simulink model "mrefrobotarm_modified_previous_y_previous_u_previous_ref_pert_2"  (R2018b)
settings: Solver=FixedStepAuto  StartTime=0.0  StopTime=60  RelTol=1e-3  AbsTol=1e-6
undefined symbols (not defined in the file or in its folder): cc, options
libraries: neural x858, simulink x1
(part 18 of 32)

== system mrefrobotarm_modified_previous_y_previous_u_previous_ref_pert_2/m=0 sd=0.2/Layer 3/Delays 1 ==
  "p{3}" : Inport  PortDimensions=30
      mask Display: e = 0.06;c1 = [120 230 180]/255;c2 = ([120 230 180]+0)/(256+128);c3 = ([120 230 180]+128)/(256+128);patch([0 1 1 0],[0 0 1 1],c1);patch([0 1 1 1-e 1-e 0+e],[0 0 1 1-e 0+e 0+e],c2);patch([0 0 1 1-e 0+e 0+e],[0 1 1 1-e 1-e 0+e],c3);plot([0 1 1 0 0],[0 0 1 1 0]);
  mux : Mux  Inputs=1
      mask Display: e = 0.06;c1 = [120 150 230]/255;c2 = ([120 150 230]+0)/383;c3 = ([120 150 230]+128)/383;patch([0 1 1 0],[0 0 1 1],c1);patch([0 1 1 1-e 1-e 0+e],[0 0 1 1-e 0+e 0+e],c2);patch([0 0 1 1-e 0+e 0+e],[0 1 1 1-e 1-e 0+e],c3);plot([0 1 1 0 0],[0 0 1 1 0]);disp('Mux')
  "pd{3,2}" : Outport
      mask Display: e = 0.06;c1 = [120 230 180]/255;c2 = ([120 230 180]+0)/(256+128);c3 = ([120 230 180]+128)/(256+128);patch([0 1 1 0],[0 0 1 1],c1);patch([0 1 1 1-e 1-e 0+e],[0 0 1 1-e 0+e 0+e],c2);patch([0 0 1 1-e 0+e 0+e],[0 1 1 1-e 1-e 0+e],c3);plot([0 1 1 0 0],[0 0 1 1 0]);
  wires:
  "p{3}"/1 -> mux/1
  mux/1 -> "pd{3,2}"/1

== system mrefrobotarm_modified_previous_y_previous_u_previous_ref_pert_2/m=0 sd=0.2/Layer 3/LW{3,2} ==
  "ad{3,2}" : Inport  PortDimensions=30
      mask Display: e = 0.06;c1 = [120 230 180]/255;c2 = ([120 230 180]+0)/(256+128);c3 = ([120 230 180]+128)/(256+128);patch([0 1 1 0],[0 0 1 1],c1);patch([0 1 1 1-e 1-e 0+e],[0 0 1 1-e 0+e 0+e],c2);patch([0 0 1 1-e 0+e 0+e],[0 1 1 1-e 1-e 0+e],c3);plot([0 1 1 0 0],[0 0 1 1 0]);
  "IW{3,2}(1,:)'" : Constant  Value=[0.0034307655937217524343141317189065375714562833309173583984375;0.0012605759437801472393203550126372647355310618877410888671875;-1.153461466440430793767291106632910668849945068359375;-0.0004563800746405328946815604940212551809963770210742950439453125;0.000423487957917458306307534332546538280439563095569610595703125;-0.6104556486794436853671186327119357883930206298828125;-0.00055692417827158009757670953376873512752354145050048828125;0.000806806139156420842710459861990557328681461513042449951171875;-0.0050279618919246947539303249641307047568261623382568359375;6.21132698530589316861239002065531167318113148212432861328125e-05;-0.0002699174804051213886861571022990347046288661658763885498046875;-0.000414437532017040803633545209549993160180747509002685546875;0.0002088822530628781852339581615041197437676601111888885498046875;-0.0001504611478212060219662726812117625740938819944858551025390625;0.0003733009737636286168478705338458212281693704426288604736328125;-0.000201439180045258521556394981644189101643860340118408203125;0.00019028402750929785509047265090742939719348214566707611083984375;0.0230900485548205490482498447590842260979115962982177734375;0.0149782123565080117766346035068636410869657993316650390625;-0.000267129024819103542444376220288404510938562452793121337890625;0.000291316583204390502394309780953562949434854090213775634765625;0.00023395696071714234924587838548859508591704070568084716796875;0.000721179756169856617416258348640667463769204914569854736328125;0.000513961448933947912497133270193216958432458341121673583984375;-0.00060880645886262946438194365583740363945253193378448486328125;-0.00022629348739984099687927443511625824612565338611602783203125;-0.00038260932582073726125615475979202528833411633968353271484375;0.0003748138698222215105249066624537590541876852512359619140625;-0.000931052496247820860451882563069148091017268598079681396484375;0.000179256690622260476432325848605842111282981932163238525390625]
      mask Display: e = 0.06;c1 = [120 150 230]/255;c2 = ([120 150 230]+0)/383;c3 = ([120 150 230]+128)/383;patch([0 1 1 0],[0 0 1 1],c1);patch([0 1 1 1-e 1-e 0+e],[0 0 1 1-e 0+e 0+e],c2);patch([0 0 1 1-e 0+e 0+e],[0 1 1 1-e 1-e 0+e],c3);plot([0 1 1 0 0],[0 0 1 1 0]);disp('weights');
  Mux : Mux  Inputs=1
      mask Display: e = 0.06;c1 = [120 150 230]/255;c2 = ([120 150 230]+0)/383;c3 = ([120 150 230]+128)/383;patch([0 1 1 0],[0 0 1 1],c1);patch([0 1 1 1-e 1-e 0+e],[0 0 1 1-e 0+e 0+e],c2);patch([0 0 1 1-e 0+e 0+e],[0 1 1 1-e 1-e 0+e],c3);plot([0 1 1 0 0],[0 0 1 1 0]);disp('Mux');
  dotprod1 : neural/Weight Functions/dotprod
  "lz{3,2}" : Outport
      mask Display: e = 0.06;c1 = [120 230 180]/255;c2 = ([120 230 180]+0)/(256+128);c3 = ([120 230 180]+128)/(256+128);patch([0 1 1 0],[0 0 1 1],c1);patch([0 1 1 1-e 1-e 0+e],[0 0 1 1-e 0+e 0+e],c2);patch([0 0 1 1-e 0+e 0+e],[0 1 1 1-e 1-e 0+e],c3);plot([0 1 1 0 0],[0 0 1 1 0]);
  wires:
  "IW{3,2}(1,:)'"/1 -> dotprod1/1
  "ad{3,2}"/1 -> dotprod1/2
  dotprod1/1 -> Mux/1
  Mux/1 -> "lz{3,2}"/1

== system mrefrobotarm_modified_previous_y_previous_u_previous_ref_pert_2/m=0 sd=0.3/Layer 1/Delays 1 ==
  "p{1}" : Inport  PortDimensions=10
      mask Display: e = 0.06;c1 = [120 230 180]/255;c2 = ([120 230 180]+0)/(256+128);c3 = ([120 230 180]+128)/(256+128);patch([0 1 1 0],[0 0 1 1],c1);patch([0 1 1 1-e 1-e 0+e],[0 0 1 1-e 0+e 0+e],c2);patch([0 0 1 1-e 0+e 0+e],[0 1 1 1-e 1-e 0+e],c3);plot([0 1 1 0 0],[0 0 1 1 0]);
  mux : Mux  Inputs=1
      mask Display: e = 0.06;c1 = [120 150 230]/255;c2 = ([120 150 230]+0)/383;c3 = ([120 150 230]+128)/383;patch([0 1 1 0],[0 0 1 1],c1);patch([0 1 1 1-e 1-e 0+e],[0 0 1 1-e 0+e 0+e],c2);patch([0 0 1 1-e 0+e 0+e],[0 1 1 1-e 1-e 0+e],c3);plot([0 1 1 0 0],[0 0 1 1 0]);disp('Mux')
  "pd{1,1}" : Outport
      mask Display: e = 0.06;c1 = [120 230 180]/255;c2 = ([120 230 180]+0)/(256+128);c3 = ([120 230 180]+128)/(256+128);patch([0 1 1 0],[0 0 1 1],c1);patch([0 1 1 1-e 1-e 0+e],[0 0 1 1-e 0+e 0+e],c2);patch([0 0 1 1-e 0+e 0+e],[0 1 1 1-e 1-e 0+e],c3);plot([0 1 1 0 0],[0 0 1 1 0]);
  wires:
  "p{1}"/1 -> mux/1
  mux/1 -> "pd{1,1}"/1

== system mrefrobotarm_modified_previous_y_previous_u_previous_ref_pert_2/m=0 sd=0.3/Layer 1/IW{1,1} ==
  "pd{1,1}" : Inport  PortDimensions=10
      mask Display: e = 0.06;c1 = [120 230 180]/255;c2 = ([120 230 180]+0)/(256+128);c3 = ([120 230 180]+128)/(256+128);patch([0 1 1 0],[0 0 1 1],c1);patch([0 1 1 1-e 1-e 0+e],[0 0 1 1-e 0+e 0+e],c2);patch([0 0 1 1-e 0+e 0+e],[0 1 1 1-e 1-e 0+e],c3);plot([0 1 1 0 0],[0 0 1 1 0]);
  "IW{1,1}(1,:)'" : Constant  Value=[-0.003130520211574626225636830412213384988717734813690185546875;-0.0267952173589505703021895755000514327548444271087646484375;0.0216826421873760437353251262493358808569610118865966796875;0.01343314188657940451421257677111498196609318256378173828125;0.03696981071744585845006980662219575606286525726318359375;0.00537900808223707414812420068983556120656430721282958984375;-0.04324594897720489272696653415550827048718929290771484375;0.0036997819464795085597774715324703720398247241973876953125;0.1522723925929859445371761239584884606301784515380859375;0.0691207001808396837017056668628356419503688812255859375]
      mask Display: e = 0.06;c1 = [120 150 230]/255;c2 = ([120 150 230]+0)/383;c3 = ([120 150 230]+128)/383;patch([0 1 1 0],[0 0 1 1],c1);patch([0 1 1 1-e 1-e 0+e],[0 0 1 1-e 0+e 0+e],c2);patch([0 0 1 1-e 0+e 0+e],[0 1 1 1-e 1-e 0+e],c3);plot([0 1 1 0 0],[0 0 1 1 0]);disp('Weights');
  "IW{1,1}(10,:)'" : Constant  Value=[-2.173041760946289979727907848428003489971160888671875;2.607292141209829328118985358742065727710723876953125;0.6405644674624635381832149505498819053173065185546875;-0.85920218141339110839993509216583333909511566162109375;-0.08361727160069791497942759406214463524520397186279296875;-1.76496085465259167079921098775230348110198974609375;1.409371438031175483018841987359337508678436279296875;-0.031758421959292737479785273535526357591152191162109375;-3.48297915503020671934564234106801450252532958984375;-3.313517995658147530235737576731480658054351806640625]
      mask Display: e = 0.06;c1 = [120 150 230]/255;c2 = ([120 150 230]+0)/383;c3 = ([120 150 230]+128)/383;patch([0 1 1 0],[0 0 1 1],c1);patch([0 1 1 1-e 1-e 0+e],[0 0 1 1-e 0+e 0+e],c2);patch([0 0 1 1-e 0+e 0+e],[0 1 1 1-e 1-e 0+e],c3);plot([0 1 1 0 0],[0 0 1 1 0]);disp('Weights');
  "IW{1,1}(11,:)'" : Constant  Value=[2.5788728163193734843616766738705337047576904296875;-1.207699405372582024398298017331399023532867431640625;-3.37948996320860128861340854200534522533416748046875;1.4627773449104939373910383437760174274444580078125;-1.0696966630890132332609709919779561460018157958984375;0.78688296052958273119060095268650911748409271240234375;0.495749525675454327799940301702008582651615142822265625;0.2432922027047803303911877037535305134952068328857421875;0.967185271859048345532983148586936295032501220703125;1.39166696149743440713564268662594258785247802734375]
      mask Display: e = 0.06;c1 = [120 150 230]/255;c2 = ([120 150 230]+0)/383;c3 = ([120 150 230]+128)/383;patch([0 1 1 0],[0 0 1 1],c1);patch([0 1 1 1-e 1-e 0+e],[0 0 1 1-e 0+e 0+e],c2);patch([0 0 1 1-e 0+e 0+e],[0 1 1 1-e 1-e 0+e],c3);plot([0 1 1 0 0],[0 0 1 1 0]);disp('Weights');
  "IW{1,1}(12,:)'" : Constant  Value=[-0.84530399280315859922296795048168860375881195068359375;2.0359030797449779726093765930272638797760009765625;-2.10702438884593590273652807809412479400634765625;1.309289253141029174543064073077403008937835693359375;1.5819124733656588777108709109597839415073394775390625;-5.56933171665802451144600127008743584156036376953125;3.706731080246947751533070913865230977535247802734375;-0.14825185642465077417995189534849487245082855224609375;-7.74086523931317049829203824629075825214385986328125;-7.437848396831068242818219005130231380462646484375]
      mask Display: e = 0.06;c1 = [120 150 230]/255;c2 = ([120 150 230]+0)/383;c3 = ([120 150 230]+128)/383;patch([0 1 1 0],[0 0 1 1],c1);patch([0 1 1 1-e 1-e 0+e],[0 0 1 1-e 0+e 0+e],c2);patch([0 0 1 1-e 0+e 0+e],[0 1 1 1-e 1-e 0+e],c3);plot([0 1 1 0 0],[0 0 1 1 0]);disp('Weights');
  "IW{1,1}(13,:)'" : Constant  Value=[-1.170619833861049396972475733491592109203338623046875;0.25194766282652547584319790985318832099437713623046875;0.52621295122762135054728105387766845524311065673828125;0.270385908341390368558876389215583913028240203857421875;1.1696880793947401766530447275727055966854095458984375;-2.4817576184281051610014401376247406005859375;1.6318379285230995012767607477144338190555572509765625;-0.2090027360255529431665166839593439362943172454833984375;-1.618597900303144765388196901767514646053314208984375;-2.462737647902751181305802674614824354648590087890625]
      mask Display: e = 0.06;c1 = [120 150 230]/255;c2 = ([120 150 230]+0)/383;c3 = ([120 150 230]+128)/383;patch([0 1 1 0],[0 0 1 1],c1);patch([0 1 1 1-e 1-e 0+e],[0 0 1 1-e 0+e 0+e],c2);patch([0 0 1 1-e 0+e 0+e],[0 1 1 1-e 1-e 0+e],c3);plot([0 1 1 0 0],[0 0 1 1 0]);disp('Weights');
  "IW{1,1}(14,:)'" : Constant  Value=[1.55110215763239267516837571747601032257080078125;-4.0823790313071270929867750965058803558349609375;3.678151929398394859305199133814312517642974853515625;0.484220240939853441286544466493069194257259368896484375;-0.299157967327123575085323636812972836196422576904296875;2.278261139134723389787495761993341147899627685546875;-1.904292313160409921835025670588947832584381103515625;-0.42705013708582006959346699659363366663455963134765625;6.1519157467350762402702457620762288570404052734375;4.12473557188791861705112751224078238010406494140625]
      mask Display: e = 0.06;c1 = [120 150 230]/255;c2 = ([120 150 230]+0)/383;c3 = ([120 150 230]+128)/383;patch([0 1 1 0],[0 0 1 1],c1);patch([0 1 1 1-e 1-e 0+e],[0 0 1 1-e 0+e 0+e],c2);patch([0 0 1 1-e 0+e 0+e],[0 1 1 1-e 1-e 0+e],c3);plot([0 1 1 0 0],[0 0 1 1 0]);disp('Weights');
  "IW{1,1}(15,:)'" : Constant  Value=[-7.49044642403462290758398012258112430572509765625;8.4556095286652688258755006245337426662445068359375;0.07683076994796754488614709543981007300317287445068359375;0.1649209519303161675107816108720726333558559417724609375;0.731078687764391332848390447907149791717529296875;0.356192025754982599661246922551072202622890472412109375;-0.70462709263987566288278685533441603183746337890625;0.454283563292785019793740275417803786695003509521484375;1.17514870947593674799236396211199462413787841796875;0.39375891485765113220196553811547346413135528564453125]
      mask Display: e = 0.06;c1 = [120 150 230]/255;c2 = ([120 150 230]+0)/383;c3 = ([120 150 230]+128)/383;patch([0 1 1 0],[0 0 1 1],c1);patch([0 1 1 1-e 1-e 0+e],[0 0 1 1-e 0+e 0+e],c2);patch([0 0 1 1-e 0+e 0+e],[0 1 1 1-e 1-e 0+e],c3);plot([0 1 1 0 0],[0 0 1 1 0]);disp('Weights');
  "IW{1,1}(16,:)'" : Constant  Value=[3.60674663571485165647345638717524707317352294921875;-2.17325942951790462842609485960565507411956787109375;0.281774062951528792009270318885683082044124603271484375;-0.46640597357186408533635813000728376209735870361328125;-0.1377159380785038245154083824672852642834186553955078125;3.641158681591715406966613954864442348480224609375;-2.97203617783390949824706694926135241985321044921875;0.398830203945743644311505704536102712154388427734375;7.51555402758171897659167370875366032123565673828125;5.60658510128899489899367836187593638896942138671875]
      mask Display: e = 0.06;c1 = [120 150 230]/255;c2 = ([120 150 230]+0)/383;c3 = ([120 150 230]+128)/383;patch([0 1 1 0],[0 0 1 1],c1);patch([0 1 1 1-e 1-e 0+e],[0 0 1 1-e 0+e 0+e],c2);patch([0 0 1 1-e 0+e 0+e],[0 1 1 1-e 1-e 0+e],c3);plot([0 1 1 0 0],[0 0 1 1 0]);disp('Weights');
  "IW{1,1}(17,:)'" : Constant  Value=[3.895626208990295769041267703869380056858062744140625;-3.943097890262982740949837534571997821331024169921875;-0.62535261500599703676783747141598723828792572021484375;0.95505929200888950436620916661922819912433624267578125;-0.383921026438908075117950602361815981566905975341796875;5.89441115817990723968478050664998590946197509765625;-4.98190169085428191664277619565837085247039794921875;-0.50685386102545992859091938953497447073459625244140625;13.2343349105093235351660041487775743007659912109375;10.3973134394820139192461283528245985507965087890625]
      mask Display: e = 0.06;c1 = [120 150 230]/255;c2 = ([120 150 230]+0)/383;c3 = ([120 150 230]+128)/383;patch([0 1 1 0],[0 0 1 1],c1);patch([0 1 1 1-e 1-e 0+e],[0 0 1 1-e 0+e 0+e],c2);patch([0 0 1 1-e 0+e 0+e],[0 1 1 1-e 1-e 0+e],c3);plot([0 1 1 0 0],[0 0 1 1 0]);disp('Weights');
  "IW{1,1}(18,:)'" : Constant  Value=[4.83070804807840659123030491173267364501953125;-4.67757984836806084416593876085244119167327880859375;0.5898717622759293011114323235233314335346221923828125;-0.70330992014694071468028369054081849753856658935546875;0.09964634194126496813392890317118144594132900238037109375;-1.9434473697030860694923148912494070827960968017578125;1.7395569293639159269559968379326164722442626953125;0.1891381389992623784923608809549477882683277130126953125;-5.341641845806972099808263010345399379730224609375;-3.855757737345567814912783433101139962673187255859375]
      mask Display: e = 0.06;c1 = [120 150 230]/255;c2 = ([120 150 230]+0)/383;c3 = ([120 150 230]+128)/383;patch([0 1 1 0],[0 0 1 1],c1);patch([0 1 1 1-e 1-e 0+e],[0 0 1 1-e 0+e 0+e],c2);patch([0 0 1 1-e 0+e 0+e],[0 1 1 1-e 1-e 0+e],c3);plot([0 1 1 0 0],[0 0 1 1 0]);disp('Weights');
  "IW{1,1}(19,:)'" : Constant  Value=[-4.59695321570936865640533142141066491603851318359375;3.10335973679891363730121156550012528896331787109375;0.7097324036484966569560128846205770969390869140625;0.36642251343099430105354485931457020342350006103515625;-0.75743674827209395150617865510866977274417877197265625;1.5712722045221225730671221754164434969425201416015625;-0.6745910287088834333957265698700211942195892333984375;-0.283992708041936048335429632061277516186237335205078125;1.6068790237467147630212593867327086627483367919921875;2.301889968806280162283428580849431455135345458984375]
      mask Display: e = 0.06;c1 = [120 150 230]/255;c2 = ([120 150 230]+0)/383;c3 = ([120 150 230]+128)/383;patch([0 1 1 0],[0 0 1 1],c1);patch([0 1 1 1-e 1-e 0+e],[0 0 1 1-e 0+e 0+e],c2);patch([0 0 1 1-e 0+e 0+e],[0 1 1 1-e 1-e 0+e],c3);plot([0 1 1 0 0],[0 0 1 1 0]);disp('Weights');
  "IW{1,1}(2,:)'" : Constant  Value=[-1.63934753678668965193310214090161025524139404296875;0.690862762150092901691778024542145431041717529296875;1.1098270396465965692556210342445410788059234619140625;-0.47701858116934847675594255633768625557422637939453125;-0.040308648879868895498201908367263968102633953094482421875;1.65398641784984334890395984984934329986572265625;-1.2211060113186926745498794844024814665317535400390625;-0.132628603903227892946148358532809652388095855712890625;4.09645662932128029609657460241578519344329833984375;3.19391469696333896166606791666708886623382568359375]
      mask Display: e = 0.06;c1 = [120 150 230]/255;c2 = ([120 150 230]+0)/383;c3 = ([120 150 230]+128)/383;patch([0 1 1 0],[0 0 1 1],c1);patch([0 1 1 1-e 1-e 0+e],[0 0 1 1-e 0+e 0+e],c2);patch([0 0 1 1-e 0+e 0+e],[0 1 1 1-e 1-e 0+e],c3);plot([0 1 1 0 0],[0 0 1 1 0]);disp('Weights');
  "IW{1,1}(20,:)'" : Constant  Value=[-2.924543314410902095090705188340507447719573974609375;2.606637417648114851687068949104286730289459228515625;0.2163646650167147245102938768468447960913181304931640625;0.1413069148377499584245953201389056630432605743408203125;-0.2152261995416087092536372438189573585987091064453125;0.61259480838460300677894565524184145033359527587890625;-0.53037461962570164875074851806857623159885406494140625;0.0188227886505173795661516322752504493109881877899169921875;0.802763207854892524295564726344309747219085693359375;0.8354223411797254694732828284031711518764495849609375]
      mask Display: e = 0.06;c1 = [120 150 230]/255;c2 = ([120 150 230]+0)/383;c3 = ([120 150 230]+128)/383;patch([0 1 1 0],[0 0 1 1],c1);patch([0 1 1 1-e 1-e 0+e],[0 0 1 1-e 0+e 0+e],c2);patch([0 0 1 1-e 0+e 0+e],[0 1 1 1-e 1-e 0+e],c3);plot([0 1 1 0 0],[0 0 1 1 0]);disp('Weights');
  "IW{1,1}(21,:)'" : Constant  Value=[1.6287518306029957759761828128830529749393463134765625;-1.0807768283750025517520043649710714817047119140625;0.74912574533584630476212851135642267763614654541015625;-1.1424226575476918998930386806023307144641876220703125;-0.0076289767086480629598721492357071838341653347015380859375;-3.021392094047862908468005116446875035762786865234375;2.358811255338060686170820190454833209514617919921875;0.0824442228272143362577395464541041292250156402587890625;-5.51327664923445670552837327704764902591705322265625;-5.30843333298950259546700181090272963047027587890625]
      mask Display: e = 0.06;c1 = [120 150 230]/255;c2 = ([120 150 230]+0)/383;c3 = ([120 150 230]+128)/383;patch([0 1 1 0],[0 0 1 1],c1);patch([0 1 1 1-e 1-e 0+e],[0 0 1 1-e 0+e 0+e],c2);patch([0 0 1 1-e 0+e 0+e],[0 1 1 1-e 1-e 0+e],c3);plot([0 1 1 0 0],[0 0 1 1 0]);disp('Weights');
  "IW{1,1}(22,:)'" : Constant  Value=[-2.15571866625504782177813467569649219512939453125;0.90437334777765132631799360751756466925144195556640625;0.9124865051952451011629818822257220745086669921875;-0.222784534930415223374922106813755817711353302001953125;0.270264179864992015733804464616696350276470184326171875;-3.276820542452375750741566662327386438846588134765625;2.530769913926180780805452741333283483982086181640625;0.236375814038352227708372765846434049308300018310546875;-5.93716416240601763121276235324330627918243408203125;-4.1254891195043938978415098972618579864501953125]
      mask Display: e = 0.06;c1 = [120 150 230]/255;c2 = ([120 150 230]+0)/383;c3 = ([120 150 230]+128)/383;patch([0 1 1 0],[0 0 1 1],c1);patch([0 1 1 1-e 1-e 0+e],[0 0 1 1-e 0+e 0+e],c2);patch([0 0 1 1-e 0+e 0+e],[0 1 1 1-e 1-e 0+e],c3);plot([0 1 1 0 0],[0 0 1 1 0]);disp('Weights');
  "IW{1,1}(23,:)'" : Constant  Value=[-10.241042556949391695297890692017972469329833984375;8.605041709768396884783214773051440715789794921875;0.116265799525851587503666451084427535533905029296875;1.419951365939454035469680093228816986083984375;1.013915460775459909115170376026071608066558837890625;-1.1869599445416458838309381462750025093555450439453125;2.03501016377486276809349874383769929409027099609375;0.5192401480506478872456455064821057021617889404296875;-5.77273799258249997734537828364409506320953369140625;-3.037495016918292822794001040165312588214874267578125]
      mask Display: e = 0.06;c1 = [120 150 230]/255;c2 = ([120 150 230]+0)/383;c3 = ([120 150 230]+128)/383;patch([0 1 1 0],[0 0 1 1],c1);patch([0 1 1 1-e 1-e 0+e],[0 0 1 1-e 0+e 0+e],c2);patch([0 0 1 1-e 0+e 0+e],[0 1 1 1-e 1-e 0+e],c3);plot([0 1 1 0 0],[0 0 1 1 0]);disp('Weights');
  "IW{1,1}(24,:)'" : Constant  Value=[4.4868037084515766110826007206924259662628173828125;-3.19150863813969909443812866811640560626983642578125;-2.318198100950282114496303620398975908756256103515625;1.5993471858336734126027067759423516690731048583984375;-0.366545935887905016681287406754563562572002410888671875;-2.558853278225889038566265298868529498577117919921875;3.08831968099624543100389928440563380718231201171875;0.043763081045771139165889707101086969487369060516357421875;-9.068107962867845373011732590384781360626220703125;-5.0355244531379117489677810226567089557647705078125]
      mask Display: e = 0.06;c1 = [120 150 230]/255;c2 = ([120 150 230]+0)/383;c3 = ([120 150 230]+128)/383;patch([0 1 1 0],[0 0 1 1],c1);patch([0 1 1 1-e 1-e 0+e],[0 0 1 1-e 0+e 0+e],c2);patch([0 0 1 1-e 0+e 0+e],[0 1 1 1-e 1-e 0+e],c3);plot([0 1 1 0 0],[0 0 1 1 0]);disp('Weights');
  "IW{1,1}(25,:)'" : Constant  Value=[-3.77232137787039079057649360038340091705322265625;2.818003452966725053130403466639108955860137939453125;1.3982425017684156909325565720791928470134735107421875;-2.707189589793884021418080010334961116313934326171875;0.3154571159197943064356195463915355503559112548828125;1.5240415822405350976254112538299523293972015380859375;-0.288077647596194086343501794544863514602184295654296875;0.340694148314549638545400966904708184301853179931640625;2.927537045689524664027203471050597727298736572265625;2.9122315337843591720456970506347715854644775390625]
      mask Display: e = 0.06;c1 = [120 150 230]/255;c2 = ([120 150 230]+0)/383;c3 = ([120 150 230]+128)/383;patch([0 1 1 0],[0 0 1 1],c1);patch([0 1 1 1-e 1-e 0+e],[0 0 1 1-e 0+e 0+e],c2);patch([0 0 1 1-e 0+e 0+e],[0 1 1 1-e 1-e 0+e],c3);plot([0 1 1 0 0],[0 0 1 1 0]);disp('Weights');
  "IW{1,1}(26,:)'" : Constant  Value=[-0.9205764108117786559404294166597537696361541748046875;1.831695246903978446795235868194140493869781494140625;1.794924319937488466081276783370412886142730712890625;-0.691656234778346590275077687692828476428985595703125;1.3900922956404431207744210041710175573825836181640625;-1.749968387145202530774668048252351582050323486328125;1.167606818024941706113395412103272974491119384765625;1.0831826655239036316658030045800842344760894775390625;0.331162905882774027954695839071064256131649017333984375;-0.2295359637529832130820039992613601498305797576904296875]
      mask Display: e = 0.06;c1 = [120 150 230]/255;c2 = ([120 150 230]+0)/383;c3 = ([120 150 230]+128)/383;patch([0 1 1 0],[0 0 1 1],c1);patch([0 1 1 1-e 1-e 0+e],[0 0 1 1-e 0+e 0+e],c2);patch([0 0 1 1-e 0+e 0+e],[0 1 1 1-e 1-e 0+e],c3);plot([0 1 1 0 0],[0 0 1 1 0]);disp('Weights');
  "IW{1,1}(27,:)'" : Constant  Value=[-8.0406385907087827291661596973426640033721923828125;7.01888963981171709605177966295741498470306396484375;-2.930376276571203586485125924809835851192474365234375;0.7645264989470923477909991561318747699260711669921875;-1.267391343179126383944321787566877901554107666015625;0.1313888970008287859769779970520175993442535400390625;1.336136338024243030986326630227267742156982421875;-0.06317770580798078017270569262109347619116306304931640625;-3.124942383741892815152141338330693542957305908203125;-1.065085108476803821275780137511901557445526123046875]
      mask Display: e = 0.06;c1 = [120 150 230]/255;c2 = ([120 150 230]+0)/383;c3 = ([120 150 230]+128)/383;patch([0 1 1 0],[0 0 1 1],c1);patch([0 1 1 1-e 1-e 0+e],[0 0 1 1-e 0+e 0+e],c2);patch([0 0 1 1-e 0+e 0+e],[0 1 1 1-e 1-e 0+e],c3);plot([0 1 1 0 0],[0 0 1 1 0]);disp('Weights');
  "IW{1,1}(28,:)'" : Constant  Value=[-0.79559927126319551771160831776796840131282806396484375;-2.4773255523127915012082667089998722076416015625;2.745290389325008906240555006661452353000640869140625;-0.77364274225923990169206945211044512689113616943359375;0.9511836511104363456325927472789771854877471923828125;5.4063895388731015856365047511644661426544189453125;-4.580760436871827323557226918637752532958984375;1.1587051139086426143620656148414127528667449951171875;6.521980450172510046513707493431866168975830078125;6.48062909794093844340068244491703808307647705078125]
      mask Display: e = 0.06;c1 = [120 150 230]/255;c2 = ([120 150 230]+0)/383;c3 = ([120 150 230]+128)/383;patch([0 1 1 0],[0 0 1 1],c1);patch([0 1 1 1-e 1-e 0+e],[0 0 1 1-e 0+e 0+e],c2);patch([0 0 1 1-e 0+e 0+e],[0 1 1 1-e 1-e 0+e],c3);plot([0 1 1 0 0],[0 0 1 1 0]);disp('Weights');
  "IW{1,1}(29,:)'" : Constant  Value=[0.9455717967309744675930005541886202991008758544921875;5.026470946769226344486014568246901035308837890625;-5.38637158776584445973867332213558256626129150390625;2.28628017314202214294027726282365620136260986328125;0.30932949189988223626102126218029297888278961181640625;-0.4933877762448501957948110430152155458927154541015625;-0.1766352589896088287613196143865934573113918304443359375;0.001762896712191657118407039916974099469371140003204345703125;0.58289944737491861115330493703368119895458221435546875;-0.20986363103695371279400205821730196475982666015625]
      mask Display: e = 0.06;c1 = [120 150 230]/255;c2 = ([120 150 230]+0)/383;c3 = ([120 150 230]+128)/383;patch([0 1 1 0],[0 0 1 1],c1);patch([0 1 1 1-e 1-e 0+e],[0 0 1 1-e 0+e 0+e],c2);patch([0 0 1 1-e 0+e 0+e],[0 1 1 1-e 1-e 0+e],c3);plot([0 1 1 0 0],[0 0 1 1 0]);disp('Weights');
  "IW{1,1}(3,:)'" : Constant  Value=[3.883665861905090110894889221526682376861572265625;-2.490540923595569555715201204293407499790191650390625;-2.0858134891025468249381447094492614269256591796875;1.7143225361438385601076106468099169433116912841796875;1.19649615017531996130628613173030316829681396484375;2.288513243747144709772101123235188424587249755859375;-2.225521935149181285140684849466197192668914794921875;-0.1395025038991163646162618761081830598413944244384765625;3.3271320187811053159521179622970521450042724609375;3.563196813572302890094078975380398333072662353515625]
      mask Display: e = 0.06;c1 = [120 150 230]/255;c2 = ([120 150 230]+0)/383;c3 = ([120 150 230]+128)/383;patch([0 1 1 0],[0 0 1 1],c1);patch([0 1 1 1-e 1-e 0+e],[0 0 1 1-e 0+e 0+e],c2);patch([0 0 1 1-e 0+e 0+e],[0 1 1 1-e 1-e 0+e],c3);plot([0 1 1 0 0],[0 0 1 1 0]);disp('Weights');
  "IW{1,1}(30,:)'" : Constant  Value=[-7.71500881523851322896234705694951117038726806640625;4.98119087929493975508421499398536980152130126953125;1.5472768291306426835518550433334894478321075439453125;-0.18501007167476080095269708181149326264858245849609375;-0.54619414331744231549947699022595770657062530517578125;4.43294788936096129106090302229858934879302978515625;-4.0094023042910720278086955659091472625732421875;-0.47923424322527707897023674377123825252056121826171875;6.95446466199350776804521956364624202251434326171875;5.82215192530926106684319165651686489582061767578125]
      mask Display: e = 0.06;c1 = [120 150 230]/255;c2 = ([120 150 230]+0)/383;c3 = ([120 150 230]+128)/383;patch([0 1 1 0],[0 0 1 1],c1);patch([0 1 1 1-e 1-e 0+e],[0 0 1 1-e 0+e 0+e],c2);patch([0 0 1 1-e 0+e 0+e],[0 1 1 1-e 1-e 0+e],c3);plot([0 1 1 0 0],[0 0 1 1 0]);disp('Weights');
  "IW{1,1}(4,:)'" : Constant  Value=[-4.64747633377341440308327946695499122142791748046875;5.4204602863823598823955762782134115695953369140625;-1.770532446384878166867338222800754010677337646484375;2.1802783676856076766625847085379064083099365234375;0.410897957606322805634846417888184078037738800048828125;-1.3650702994955865587911603142856620252132415771484375;0.9995539007256677432877722822013311088085174560546875;0.019136215359868459506831328553744242526590824127197265625;-2.668794373156969879090638642082922160625457763671875;-2.98555660082689922063536869245581328868865966796875]
      mask Display: e = 0.06;c1 = [120 150 230]/255;c2 = ([120 150 230]+0)/383;c3 = ([120 150 230]+128)/383;patch([0 1 1 0],[0 0 1 1],c1);patch([0 1 1 1-e 1-e 0+e],[0 0 1 1-e 0+e 0+e],c2);patch([0 0 1 1-e 0+e 0+e],[0 1 1 1-e 1-e 0+e],c3);plot([0 1 1 0 0],[0 0 1 1 0]);disp('Weights');
  "IW{1,1}(5,:)'" : Constant  Value=[-0.8128589299221917752191757244872860610485076904296875;3.065173803821313214257315848954021930694580078125;-3.417192646381593146287514173309318721294403076171875;0.080156680002492375347600273016723804175853729248046875;0.151590970284561976644255310020525939762592315673828125;0.018025384289908040480465700738932355307042598724365234375;-0.313673696104543708873535479142447002232074737548828125;-0.1791878297053093593849126818895456381142139434814453125;1.850426685418060213095259314286522567272186279296875;0.7836020987121390390939268399961292743682861328125]
      mask Display: e = 0.06;c1 = [120 150 230]/255;c2 = ([120 150 230]+0)/383;c3 = ([120 150 230]+128)/383;patch([0 1 1 0],[0 0 1 1],c1);patch([0 1 1 1-e 1-e 0+e],[0 0 1 1-e 0+e 0+e],c2);patch([0 0 1 1-e 0+e 0+e],[0 1 1 1-e 1-e 0+e],c3);plot([0 1 1 0 0],[0 0 1 1 0]);disp('Weights');
  "IW{1,1}(6,:)'" : Constant  Value=[-4.271610147259554679521897924132645130157470703125;0.2375953752669804630581751325735240243375301361083984375;1.0537049904606539119100716561661101877689361572265625;2.518695607995106389154216230963356792926788330078125;0.338311306850040072191632134490646421909332275390625;-6.55703521381559095715374496649019420146942138671875;5.08303328675847776452201287611387670040130615234375;-0.279403585733045523031847778838709928095340728759765625;-11.601407660281996214735045214183628559112548828125;-12.365652046129394392437461647205054759979248046875]
      mask Display: e = 0.06;c1 = [120 150 230]/255;c2 = ([120 150 230]+0)/383;c3 = ([120 150 230]+128)/383;patch([0 1 1 0],[0 0 1 1],c1);patch([0 1 1 1-e 1-e 0+e],[0 0 1 1-e 0+e 0+e],c2);patch([0 0 1 1-e 0+e 0+e],[0 1 1 1-e 1-e 0+e],c3);plot([0 1 1 0 0],[0 0 1 1 0]);disp('Weights');
  "IW{1,1}(7,:)'" : Constant  Value=[4.51972036193820247973462755908258259296417236328125;-1.8187936004655977928479160254937596619129180908203125;-1.0502068932096670916820357888354919850826263427734375;-0.8259581577950940722843142793863080441951751708984375;-1.1454534391080624100567320056143216788768768310546875;2.219426997983873661723919212818145751953125;-1.1959267654694205607057710949447937309741973876953125;0.260162923182675864808288679341785609722137451171875;0.296506517546240078164743181332596577703952789306640625;1.7390611930111747884808437447645701467990875244140625]
      mask Display: e = 0.06;c1 = [120 150 230]/255;c2 = ([120 150 230]+0)/383;c3 = ([120 150 230]+128)/383;patch([0 1 1 0],[0 0 1 1],c1);patch([0 1 1 1-e 1-e 0+e],[0 0 1 1-e 0+e 0+e],c2);patch([0 0 1 1-e 0+e 0+e],[0 1 1 1-e 1-e 0+e],c3);plot([0 1 1 0 0],[0 0 1 1 0]);disp('Weights');
  "IW{1,1}(8,:)'" : Constant  Value=[-0.55034633025198009814715760512626729905605316162109375;-0.104595256493204669112628835137002170085906982421875;0.8971406404050428218255319734453223645687103271484375;0.08822992584952100980633105109518510289490222930908203125;0.25000840933475576566280551560339517891407012939453125;0.51447958402818461109973213751800358295440673828125;-0.62833701148975340533553435307112522423267364501953125;-0.0170619164647444025717515359019671450369060039520263671875;2.167617608052587296896263069356791675090789794921875;1.3205119745454723112487727121333591639995574951171875]
      mask Display: e = 0.06;c1 = [120 150 230]/255;c2 = ([120 150 230]+0)/383;c3 = ([120 150 230]+128)/383;patch([0 1 1 0],[0 0 1 1],c1);patch([0 1 1 1-e 1-e 0+e],[0 0 1 1-e 0+e 0+e],c2);patch([0 0 1 1-e 0+e 0+e],[0 1 1 1-e 1-e 0+e],c3);plot([0 1 1 0 0],[0 0 1 1 0]);disp('Weights');
  "IW{1,1}(9,:)'" : Constant  Value=[7.5101382209504397025057187420316040515899658203125;-6.1401063903558910084257149719633162021636962890625;-1.223586239650691798175330404774285852909088134765625;1.441957950449608727438999267178587615489959716796875;-0.256070145143549698918405965741840191185474395751953125;5.157489996400091314399105613119900226593017578125;-3.715554304611389913048924427130259573459625244140625;-0.043874413895675166974452707790987915359437465667724609375;8.935515118645042775824549607932567596435546875;6.887353805857657107480918057262897491455078125]
      mask Display: e = 0.06;c1 = [120 150 230]/255;c2 = ([120 150 230]+0)/383;c3 = ([120 150 230]+128)/383;patch([0 1 1 0],[0 0 1 1],c1);patch([0 1 1 1-e 1-e 0+e],[0 0 1 1-e 0+e 0+e],c2);patch([0 0 1 1-e 0+e 0+e],[0 1 1 1-e 1-e 0+e],c3);plot([0 1 1 0 0],[0 0 1 1 0]);disp('Weights');
  Mux : Mux  Inputs=30
      mask Display: e = 0.06;c1 = [120 150 230]/255;c2 = ([120 150 230]+0)/383;c3 = ([120 150 230]+128)/383;patch([0 1 1 0],[0 0 1 1],c1);patch([0 1 1 1-e 1-e 0+e],[0 0 1 1-e 0+e 0+e],c2);patch([0 0 1 1-e 0+e 0+e],[0 1 1 1-e 1-e 0+e],c3);plot([0 1 1 0 0],[0 0 1 1 0]);disp('Mux');
  dotprod{1..30} (30 alike) : neural/Weight Functions/dotprod
  "iz{1,1}" : Outport
      mask Display: e = 0.06;c1 = [120 230 180]/255;c2 = ([120 230 180]+0)/(256+128);c3 = ([120 230 180]+128)/(256+128);patch([0 1 1 0],[0 0 1 1],c1);patch([0 1 1 1-e 1-e 0+e],[0 0 1 1-e 0+e 0+e],c2);patch([0 0 1 1-e 0+e 0+e],[0 1 1 1-e 1-e 0+e],c3);plot([0 1 1 0 0],[0 0 1 1 0]);
  wires:
  "IW{1,1}(1,:)'"/1 -> dotprod1/1
  "pd{1,1}"/1 -> dotprod1/2, dotprod2/2, dotprod3/2, dotprod4/2, dotprod5/2, dotprod6/2, dotprod7/2, dotprod8/2, dotprod9/2, dotprod10/2, dotprod11/2, dotprod12/2, dotprod13/2, dotprod14/2, dotprod15/2, dotprod16/2, dotprod17/2, dotprod18/2, dotprod19/2, dotprod20/2, dotprod21/2, dotprod22/2, dotprod23/2, dotprod24/2, dotprod25/2, dotprod26/2, dotprod27/2, dotprod28/2, dotprod29/2, dotprod30/2
  dotprod1/1 -> Mux/1
  "IW{1,1}(2,:)'"/1 -> dotprod2/1
  dotprod2/1 -> Mux/2
  "IW{1,1}(3,:)'"/1 -> dotprod3/1
  dotprod3/1 -> Mux/3
  "IW{1,1}(4,:)'"/1 -> dotprod4/1
  dotprod4/1 -> Mux/4
  "IW{1,1}(5,:)'"/1 -> dotprod5/1
  dotprod5/1 -> Mux/5
  "IW{1,1}(6,:)'"/1 -> dotprod6/1
  dotprod6/1 -> Mux/6
  "IW{1,1}(7,:)'"/1 -> dotprod7/1
  dotprod7/1 -> Mux/7
  "IW{1,1}(8,:)'"/1 -> dotprod8/1
  dotprod8/1 -> Mux/8
  "IW{1,1}(9,:)'"/1 -> dotprod9/1
  dotprod9/1 -> Mux/9
  "IW{1,1}(10,:)'"/1 -> dotprod10/1
  dotprod10/1 -> Mux/10
  "IW{1,1}(11,:)'"/1 -> dotprod11/1
  dotprod11/1 -> Mux/11
  "IW{1,1}(12,:)'"/1 -> dotprod12/1
  dotprod12/1 -> Mux/12
  "IW{1,1}(13,:)'"/1 -> dotprod13/1
  dotprod13/1 -> Mux/13
  "IW{1,1}(14,:)'"/1 -> dotprod14/1
  dotprod14/1 -> Mux/14
  "IW{1,1}(15,:)'"/1 -> dotprod15/1
  dotprod15/1 -> Mux/15
  "IW{1,1}(16,:)'"/1 -> dotprod16/1
  dotprod16/1 -> Mux/16
  "IW{1,1}(17,:)'"/1 -> dotprod17/1
  dotprod17/1 -> Mux/17
  "IW{1,1}(18,:)'"/1 -> dotprod18/1
  dotprod18/1 -> Mux/18
  "IW{1,1}(19,:)'"/1 -> dotprod19/1
  dotprod19/1 -> Mux/19
  "IW{1,1}(20,:)'"/1 -> dotprod20/1
  dotprod20/1 -> Mux/20
  "IW{1,1}(21,:)'"/1 -> dotprod21/1
  dotprod21/1 -> Mux/21
  "IW{1,1}(22,:)'"/1 -> dotprod22/1
  dotprod22/1 -> Mux/22
  "IW{1,1}(23,:)'"/1 -> dotprod23/1
  dotprod23/1 -> Mux/23
  "IW{1,1}(24,:)'"/1 -> dotprod24/1
  dotprod24/1 -> Mux/24
  "IW{1,1}(25,:)'"/1 -> dotprod25/1
  dotprod25/1 -> Mux/25
  "IW{1,1}(26,:)'"/1 -> dotprod26/1
  dotprod26/1 -> Mux/26
  "IW{1,1}(27,:)'"/1 -> dotprod27/1
  dotprod27/1 -> Mux/27
  "IW{1,1}(28,:)'"/1 -> dotprod28/1
  dotprod28/1 -> Mux/28
  "IW{1,1}(29,:)'"/1 -> dotprod29/1
  dotprod29/1 -> Mux/29
  "IW{1,1}(30,:)'"/1 -> dotprod30/1
  dotprod30/1 -> Mux/30
  Mux/1 -> "iz{1,1}"/1

== system mrefrobotarm_modified_previous_y_previous_u_previous_ref_pert_2/m=0 sd=0.3/Layer 2/Delays 1 ==
  "p{2}" : Inport  PortDimensions=30
      mask Display: e = 0.06;c1 = [120 230 180]/255;c2 = ([120 230 180]+0)/(256+128);c3 = ([120 230 180]+128)/(256+128);patch([0 1 1 0],[0 0 1 1],c1);patch([0 1 1 1-e 1-e 0+e],[0 0 1 1-e 0+e 0+e],c2);patch([0 0 1 1-e 0+e 0+e],[0 1 1 1-e 1-e 0+e],c3);plot([0 1 1 0 0],[0 0 1 1 0]);
  mux : Mux  Inputs=1
      mask Display: e = 0.06;c1 = [120 150 230]/255;c2 = ([120 150 230]+0)/383;c3 = ([120 150 230]+128)/383;patch([0 1 1 0],[0 0 1 1],c1);patch([0 1 1 1-e 1-e 0+e],[0 0 1 1-e 0+e 0+e],c2);patch([0 0 1 1-e 0+e 0+e],[0 1 1 1-e 1-e 0+e],c3);plot([0 1 1 0 0],[0 0 1 1 0]);disp('Mux')
  "pd{2,1}" : Outport
      mask Display: e = 0.06;c1 = [120 230 180]/255;c2 = ([120 230 180]+0)/(256+128);c3 = ([120 230 180]+128)/(256+128);patch([0 1 1 0],[0 0 1 1],c1);patch([0 1 1 1-e 1-e 0+e],[0 0 1 1-e 0+e 0+e],c2);patch([0 0 1 1-e 0+e 0+e],[0 1 1 1-e 1-e 0+e],c3);plot([0 1 1 0 0],[0 0 1 1 0]);
  wires:
  "p{2}"/1 -> mux/1
  mux/1 -> "pd{2,1}"/1
